simulink model "ASR_OpenLoop"  (R2019b)
settings: Solver=ode5  StartTime=0.0  StopTime=12  FixedStep=T_Step  RelTol=1e-3
values from neighbouring files (symbols this model uses):
  a = 1    [ASR_OpenLoop_Properties.m]
  alpha_1 = -pi/2    (= -1.57079632679)    [ASR_OpenLoop_Properties.m]
  alpha_2 = -1    [ASR_OpenLoop_Properties.m]
  alpha_3 = 2    [ASR_OpenLoop_Properties.m]
  beta_1 = 0    [ASR_OpenLoop_Properties.m]
  beta_2 = -pi/(4*alpha_2)    (= 0.785398163397)    [ASR_OpenLoop_Properties.m]
  beta_3 = (3.6365*pi^2) / (2*alpha_3^2)    (= 4.48635205057)    [ASR_OpenLoop_Properties.m]
  c0 = c(1)    [ASR_OpenLoop_Properties.m]
  c1 = c(2)    [ASR_OpenLoop_Properties.m]
  c2 = c(3)    [ASR_OpenLoop_Properties.m]
  Input_Selector = 3    [ASR_OpenLoop_Properties.m]
  N_Int = 3    [ASR_OpenLoop_Properties.m]
  P_u1 = x_final - x_init / T_Total    (= -0.333333333333)    [ASR_OpenLoop_Properties.m]
  PC_u1_1 = (x_final - x_init) / T_Total    (= -0.333333333333)    [ASR_OpenLoop_Properties.m]
  PC_u1_2 = PC_u1_1    (= -0.333333333333)    [ASR_OpenLoop_Properties.m]
  PC_u1_3 = PC_u1_1    (= -0.333333333333)    [ASR_OpenLoop_Properties.m]
  PC_u2_1 = 0.2344    [ASR_OpenLoop_Properties.m]
  PC_u2_2 = -0.2812    [ASR_OpenLoop_Properties.m]
  PC_u2_3 = 0.0469    [ASR_OpenLoop_Properties.m]
  phi_init = pi/4    (= 0.785398163397)    [ASR_OpenLoop_Properties.m]
  psi_init = 0    [ASR_OpenLoop_Properties.m]
  T_Int = 12/N_Int    (= 4)    [ASR_OpenLoop_Properties.m]
  w = 2*pi/T_Int    (= 1.57079632679)    [ASR_OpenLoop_Properties.m]
  x_init = 4    [ASR_OpenLoop_Properties.m]
  y_init = 1    [ASR_OpenLoop_Properties.m]
libraries: simulink x1
settings Model: Creator=kerrm  LastModifiedBy=kerrm
settings DataIOCC: ReturnWorkspaceOutputs=off

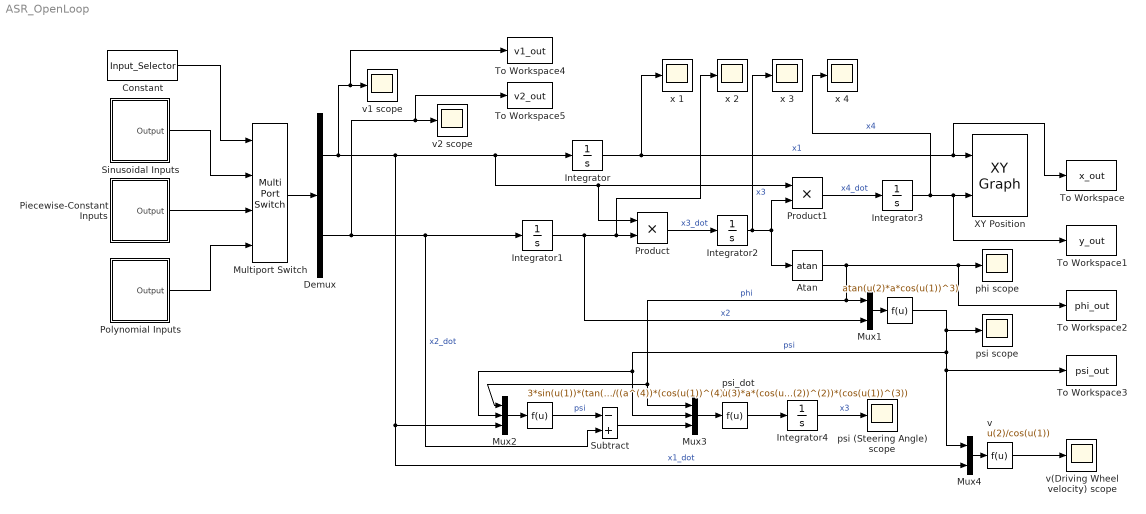
== system ASR_OpenLoop ==
  " " : Fcn  Expr=atan(u(2)*a*cos(u(1))^3)
  " " : Fcn  Expr=3*sin(u(1))*(tan(u(2))^(2))*u(3)/((a^(4))*(cos(u(1))^(4)))
  Atan : Trigonometry  Operator=atan
  Constant : Constant  Value=Input_Selector
  Demux : Demux  Outputs=2
  Integrator : Integrator  InitialCondition=x_init
  Integrator1 : Integrator  InitialCondition=tan(psi_init)/(a*cos(phi_init)^3)
  Integrator2 : Integrator  InitialCondition=tan(phi_init)
  Integrator3 : Integrator  InitialCondition=y_init
  Integrator4 : Integrator  InitialCondition=psi_init
  Multiport Switch : MultiPortSwitch
  Mux1 : Mux  Inputs=2
  Mux2 : Mux  Inputs=3
  Mux3 : Mux  Inputs=3
  Mux4 : Mux  Inputs=2
  Piecewise-Constant Inputs : Subsystem
  Polynomial Inputs : Subsystem
  Product : Product
  Product1 : Product
  Sinusoidal Inputs : Subsystem
  Subtract : Sum  Inputs=-+
  To Workspace : ToWorkspace  VariableName=x_out  SaveFormat=Timeseries  SampleTime=-1
  To Workspace1 : ToWorkspace  VariableName=y_out  SaveFormat=Timeseries  SampleTime=-1
  To Workspace2 : ToWorkspace  VariableName=phi_out  SaveFormat=Timeseries  SampleTime=-1
  To Workspace3 : ToWorkspace  VariableName=psi_out  SaveFormat=Timeseries  SampleTime=-1
  To Workspace4 : ToWorkspace  VariableName=v1_out  SaveFormat=Timeseries  SampleTime=-1
  To Workspace5 : ToWorkspace  VariableName=v2_out  SaveFormat=Timeseries  SampleTime=-1
  "XY Position " : simulink/Sinks/XY Graph  xmin=-5  xmax=5  ymin=-5  ymax=5  st=-1
  phi scope : Scope
  psi (Steering Angle) scope : Scope
  psi scope : Scope
  "psi_dot " : Fcn  Expr=u(3)*a*(cos(u(2))^(2))*(cos(u(1))^(3))
  v : Fcn  Expr=u(2)/cos(u(1))
  v(Driving Wheel velocity) scope : Scope
  v1 scope : Scope
  v2 scope : Scope
  x {1..4} (4 alike) : Scope
  wires:
  Demux/1 -> Mux2/3, Mux4/2, Product1/1, Product/1, Integrator/1, To Workspace4/1, v1 scope/1  "x1_dot"
  Integrator/1 -> x 1/1, To Workspace/1, "XY Position "/1  "x1"
  Demux/2 -> Subtract/2, Integrator1/1, To Workspace5/1, v2 scope/1  "x2_dot"
  Integrator1/1 -> Mux1/2, x 2/1, Product/2  "x2"
  Product/1 -> Integrator2/1  "x3_dot"
  Integrator2/1 -> x 3/1, Atan/1, Product1/2  "x3"
  Product1/1 -> Integrator3/1  "x4_dot"
  Integrator3/1 -> x 4/1, To Workspace1/1, "XY Position "/2  "x4"
  Atan/1 -> To Workspace2/1, phi scope/1, Mux3/1, Mux2/1, Mux1/1  "phi"
  " "/1 -> psi scope/1, To Workspace3/1, Mux4/1, Mux3/2, Mux2/2  "psi"
  Mux1/1 -> " "/1
  Piecewise-Constant Inputs/1(Output) -> Multiport Switch/3
  Constant/1 -> Multiport Switch/1
  Multiport Switch/1 -> Demux/1
  Sinusoidal Inputs/1(Output) -> Multiport Switch/2
  Polynomial Inputs/1(Output) -> Multiport Switch/4
  Mux2/1 -> " "/1
  " "/1 -> Subtract/1  "psi"
  Subtract/1 -> Mux3/3
  Mux3/1 -> "psi_dot "/1
  "psi_dot "/1 -> Integrator4/1
  Integrator4/1 -> psi (Steering Angle) scope/1  "x3"
  Mux4/1 -> v/1
  v/1 -> v(Driving Wheel velocity) scope/1

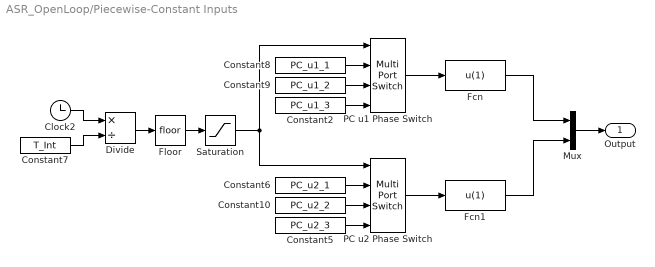
== system ASR_OpenLoop/Piecewise-Constant Inputs ==
  Clock2 : Clock
  Constant10 : Constant  Value=PC_u2_2  VectorParams1D=off
  Constant2 : Constant  Value=PC_u1_3  VectorParams1D=off
  Constant5 : Constant  Value=PC_u2_3  VectorParams1D=off
  Constant6 : Constant  Value=PC_u2_1
  Constant7 : Constant  Value=T_Int
  Constant8 : Constant  Value=PC_u1_1
  Constant9 : Constant  Value=PC_u1_2  VectorParams1D=off
  Divide : Product  Inputs=*/
  Fcn : Fcn  Expr=u(1)
  Fcn1 : Fcn  Expr=u(1)
  Floor : Rounding
  Mux : Mux  Inputs=2
  PC u1 Phase Switch : MultiPortSwitch  DataPortOrder=Zero-based contiguous  DiagnosticForDefault=None  zeroidx=on
  PC u2 Phase Switch : MultiPortSwitch  DataPortOrder=Zero-based contiguous  DiagnosticForDefault=None  zeroidx=on
  Saturation : Saturate  UpperLimit=N_Int - 1  LowerLimit=0
  Output : Outport
  wires:
  Constant10/1 -> PC u2 Phase Switch/3
  Fcn1/1 -> Mux/2
  PC u2 Phase Switch/1 -> Fcn1/1
  Saturation/1 -> PC u1 Phase Switch/1, PC u2 Phase Switch/1
  Fcn/1 -> Mux/1
  Floor/1 -> Saturation/1
  Constant8/1 -> PC u1 Phase Switch/2
  Constant9/1 -> PC u1 Phase Switch/3
  Constant5/1 -> PC u2 Phase Switch/4
  Clock2/1 -> Divide/1
  PC u1 Phase Switch/1 -> Fcn/1
  Constant7/1 -> Divide/2
  Mux/1 -> Output/1
  Divide/1 -> Floor/1
  Constant2/1 -> PC u1 Phase Switch/4
  Constant6/1 -> PC u2 Phase Switch/2

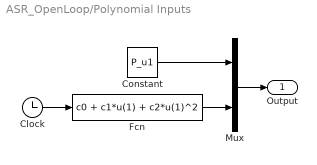
== system ASR_OpenLoop/Polynomial Inputs ==
  Clock : Clock
  Constant : Constant  Value=P_u1
  Fcn : Fcn  Expr=c0 + c1*u(1) + c2*u(1)^2
  Mux : Mux  Inputs=2
  Output : Outport
  wires:
  Mux/1 -> Output/1
  Constant/1 -> Mux/1
  Clock/1 -> Fcn/1
  Fcn/1 -> Mux/2

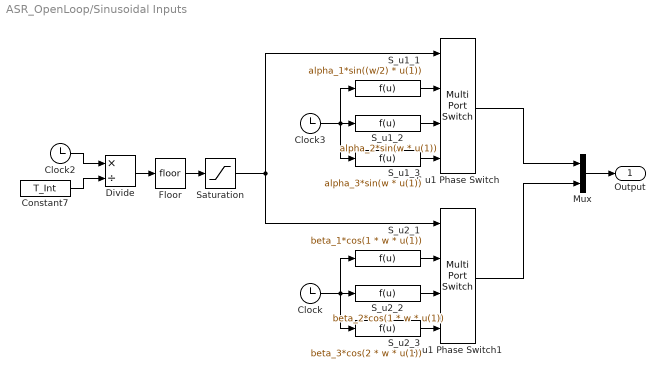
== system ASR_OpenLoop/Sinusoidal Inputs ==
  Clock : Clock
  Clock2 : Clock
  Clock3 : Clock
  Constant7 : Constant  Value=T_Int
  Divide : Product  Inputs=*/
  Floor : Rounding
  Mux : Mux  Inputs=2
  S u1 Phase Switch : MultiPortSwitch  DataPortOrder=Zero-based contiguous  DiagnosticForDefault=None  zeroidx=on
  S u1 Phase Switch1 : MultiPortSwitch  DataPortOrder=Zero-based contiguous  DiagnosticForDefault=None  zeroidx=on
  S_u1_1 : Fcn  Expr=alpha_1*sin((w/2) * u(1))
  S_u1_2 : Fcn  Expr=alpha_2*sin(w * u(1))
  S_u1_3 : Fcn  Expr=alpha_3*sin(w * u(1))
  S_u2_1 : Fcn  Expr=beta_1*cos(1 * w * u(1))
  S_u2_2 : Fcn  Expr=beta_2*cos(1 * w * u(1))
  S_u2_3 : Fcn  Expr=beta_3*cos(2 * w * u(1))
  Saturation : Saturate  UpperLimit=N_Int - 1  LowerLimit=0
  Output : Outport
  wires:
  Constant7/1 -> Divide/2
  Divide/1 -> Floor/1
  S u1 Phase Switch/1 -> Mux/1
  Clock2/1 -> Divide/1
  Floor/1 -> Saturation/1
  S u1 Phase Switch1/1 -> Mux/2
  Mux/1 -> Output/1
  Saturation/1 -> S u1 Phase Switch1/1, S u1 Phase Switch/1
  S_u1_1/1 -> S u1 Phase Switch/2
  Clock3/1 -> S_u1_1/1, S_u1_2/1, S_u1_3/1
  S_u1_2/1 -> S u1 Phase Switch/3
  S_u1_3/1 -> S u1 Phase Switch/4
  S_u2_3/1 -> S u1 Phase Switch1/4
  S_u2_2/1 -> S u1 Phase Switch1/3
  S_u2_1/1 -> S u1 Phase Switch1/2
  Clock/1 -> S_u2_1/1, S_u2_2/1, S_u2_3/1
